simulink subsystem "Controller"  (R2020b)
settings: Solver=VariableStepAuto  StartTime=0.0  StopTime=10.0  RelTol=1e-3
values from neighbouring files (symbols this model uses):
  alpha = 0.5    [scratch.m]    (also in startup.m = 0.9)
  B = [-1,  0, 0, 0 ... (first row only)    [startup.m]
  g = 9.80665    [startup.m]
  leg_length = 1    [startup.m]
  leg_mass = 1.0    (= 1)    [startup.m]
  theta3_ref = -pi/4    (= -0.785398163397)    [scratch.m]    (also in startup.m = 0.785398163397)
  torso_length = 0.6    [startup.m]
  torso_mass = 1.0    (= 1)    [startup.m]
settings Model: Creator=PaulWintz  LastModifiedBy=PaulWintz

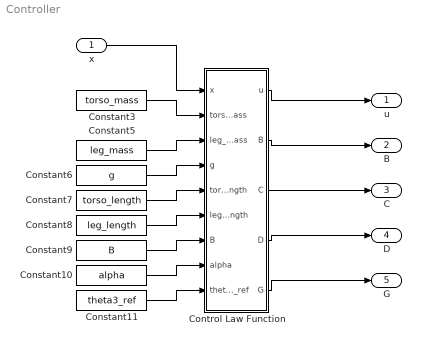
== system Controller ==
  x : Inport
  Constant10 : Constant  Value=alpha
  Constant11 : Constant  Value=theta3_ref
  Constant3 : Constant  Value=torso_mass
  Constant5 : Constant  Value=leg_mass
  Constant6 : Constant  Value=g
  Constant7 : Constant  Value=torso_length
  Constant8 : Constant  Value=leg_length
  Constant9 : Constant  Value=B
  Control Law Function : MATLAB Function  TreatAsAtomicUnit=on
  u : Outport
  B : Outport  Port=2
  C : Outport  Port=3
  D : Outport  Port=4
  G : Outport  Port=5
  wires:
  Constant10/1 -> Control Law Function/8(alpha)
  Constant3/1 -> Control Law Function/2(torso_mass)
  Constant6/1 -> Control Law Function/4(g)
  x/1 -> Control Law Function/1(x)
  Constant11/1 -> Control Law Function/9(theta3_ref)
  Constant5/1 -> Control Law Function/3(leg_mass)
  Constant7/1 -> Control Law Function/5(torso_length)
  Constant8/1 -> Control Law Function/6(leg_length)
  Constant9/1 -> Control Law Function/7("B ")
  Control Law Function/4(D) -> D/1
  Control Law Function/3(C) -> C/1
  Control Law Function/2(B) -> B/1
  Control Law Function/5(G) -> G/1
  Control Law Function/1(u) -> u/1

== matlab function Controller/Control Law Function ==
  settings: updateMethod=DISCRETE
  data: x input size=10; torso_mass input; u output; leg_mass input; g input; torso_length input; leg_length input; B input; alpha input; theta3_ref input; B output; C output; D output; G output
function [u, B, C, D, G] = control_law(x, torso_mass, leg_mass, g, torso_length, leg_length, B, alpha, theta3_ref)

    theta1 = x(1);
    theta2 = x(2);
    theta3 = x(3);
    theta4 = x(4);
    theta5 = x(5);
    omega1 = x(6);
    omega2 = x(7);
    omega3 = x(8);
    omega4 = x(9);
    omega5 = x(10);
    omega = x(6:10);
    
    m1 = leg_mass; %m1_sig
    m2 = leg_mass; %m2_sig
    m3 = leg_mass; %m3_sig
    m4 = leg_mass; %m4_sig
    m5 = torso_mass; %m5_sig
    
    L1 = leg_length; %L1_sig
    L2 = leg_length; %L2_sig
    L3 = leg_length; %L3_sig
    L4 = leg_length; %L4_sig
    L5 = torso_length; %L5_sig
  
    H = [1 0 0 0 0; 
         0 1 0 0 0; 
         0 0 1 0 0; 
         0 0 0 0 1];

    %hip_mass_sig is removed from the parameters of dynamic_matrices
    [C, D, G] = dynamic_matrices(x, g, torso_mass, leg_mass, leg_length, torso_length);

    y = [theta1;
        theta2;
        theta3-theta3_ref;
        theta5];
    Lf = [omega1; 
          omega2; 
          omega3; 
          omega5]; 
    LfLf = H * (D \ (-C*omega - G));
    LgLf = H * (D \ B);

    ydot = Lf;

    Psi = [psi_f([y(1); ydot(1)], alpha); 
           psi_f([y(2); ydot(2)], alpha); 
           psi_f([y(3); ydot(3)], alpha); 
           psi_f([y(4); ydot(4)], alpha)];
    u = LgLf \ (Psi - LfLf);

end

function y = phi(x, alpha_sig)
    y = x(1) + (1/2 - alpha_sig)*sign(x(2)).*abs(x(2)).^(2 - alpha_sig);
end

function y = psi_f(x, alpha_sig)
     y = -sign(x(2)).*abs(x(2)).^alpha_sig - sign(phi(x, alpha_sig)).*abs(phi(x, alpha_sig)).^(alpha_sig/(2-alpha_sig));
end

function [C, D, G] = dynamic_matrices(x, g, torso_mass, leg_mass, leg_length, torso_length)
                    %m1_sig, m2_sig, m3_sig, m4_sig, m5_sig, L1_sig, L2_sig, L3_sig, L4_sig, L5_sig

    theta1 = x(1);
    theta2 = x(2);
    theta3 = x(3);
    theta4 = x(4);
    theta5 = x(5);
    omega1 = x(6);
    omega2 = x(7);
    omega3 = x(8);
    omega4 = x(9);
    omega5 = x(10);
    
    %
    alpha10 = theta1;
    alpha20 = alpha10+theta2;
    alpha30 = alpha20+theta3;
    alpha40 = alpha30+theta4;
    alpha50 = alpha40+theta5;
    
    alpha21 = theta2;
    alpha31 = alpha21+theta3;
    alpha41 = alpha31+theta4;
    alpha51 = alpha21+theta5;
    
    alpha12 = -alpha21;
    alpha32 = theta3;
    alpha42 = alpha32+theta4;
    alpha52 = theta5;
    
    alpha13 = -alpha31;
    alpha23 = -alpha32;
    alpha43 = theta4;
    
    alpha14 = -alpha41;
    alpha24 = -alpha42;
    alpha34 = -alpha43;
    
    alpha15 = -alpha51;
    alpha25 = -alpha52;
    
    %R_22 = cos()
    
    R10_22 = cos(alpha10);
    R20_22 = cos(alpha20); 
    R30_22 = cos(alpha30); 
    R40_22 = cos(alpha40);
    R50_22 = cos(alpha50);
    
    R21_22 = cos(alpha21);
    R31_22 = cos(alpha31);
    R41_22 = cos(alpha41);
    R51_22 = cos(alpha51);
    
    R12_22 = cos(alpha12);
    R32_22 = cos(alpha32);
    R42_22 = cos(alpha42);
    R52_22 = cos(alpha52);
    
    R13_22 = cos(alpha13);
    R23_22 = cos(alpha23);
    R43_22 = cos(alpha43);
    
    R14_22 = cos(alpha14);
    R24_22 = cos(alpha24);
    R34_22 = cos(alpha34);
    
    R15_22 = cos(alpha15);
    R25_22 = cos(alpha25);
    
    %R_21 = sin()
    R21_21 = sin(alpha21);
    R31_21 = sin(alpha31);
    R41_21 = sin(alpha41);
    R51_21 = sin(alpha51);
    
    R12_21 = sin(alpha12);
    R32_21 = sin(alpha32);
    R42_21 = sin(alpha42);
    R52_21 = sin(alpha52);
    
    R13_21 = sin(alpha13);
    R23_21 = sin(alpha23);
    R43_21 = sin(alpha43);
    
    R14_21 = sin(alpha14);
    R24_21 = sin(alpha24);
    R34_21 = sin(alpha34);
    
    R15_21 = sin(alpha15);
    R25_21 = sin(alpha25);
    
    %I defined the masses and lengths in terms of leg_mass and
    %leg_length because they're already defined
    m1 = leg_mass; %m1_sig
    m2 = leg_mass; %m2_sig
    m3 = leg_mass; %m3_sig
    m4 = leg_mass; %m4_sig
    m5 = torso_mass; %m5_sig
    
    L1 = leg_length; %L1_sig
    L2 = leg_length; %L2_sig
    L3 = leg_length; %L3_sig
    L4 = leg_length; %L4_sig
    L5 = torso_length; %L5_sig   
    
    Pi = [(m1/4)+m2+m3+m4+m5, (m2+m3+m4+m5)*R12_22, (m3+m4)*R13_22, m4*R14_22, m5*R15_22;
        ((m2/2)+m3+m4+m5)*R21_22, m2/4+m3+m4+m5, (m3+m4)*R23_22, m4*R24_22, m5*R25_22;
        ((m3/2)+m4)*R31_22, ((m3/2)+m4)*R32_22, (m3/4)+m4, m4*R34_22, 0;
        m4/2*R41_22, m4/2*R42_22, m4/2*R43_22, m4/4, 0;
        m5/2*R51_22, m5/2*R52_22, 0, 0, m5/2];
    
    Lambda = [0, (m2+m3+m4+m5)*R12_21, (m3+m4)*R13_21, m4*R14_21, m5*R15_21;
        ((m2/2)+m3+m4+m5)*R21_21, 0, (m3+m4)*R23_21, m4*R24_21, m5*R25_21;
        ((m3/2)+m4)*R31_21, ((m3/2)+m4)*R32_21, 0, m4*R34_21, 0;
        m4/2*R41_21, m4/2*R42_21, m4/2*R43_21, 0, 0;
        m5/2*R51_21, m5/2*R52_21, 0, 0, 0];
    
    L = diag([L1, L2, L3, L4, L5]);
    
    G = g*[L1*(3/2*m1+m2+m3+m4+m5)*R10_22;
        L2*(3/2*m2+m3+m4+m5)*R20_22;
        L3*(3/2*m3+m4)*R30_22;
        3/2*L4*m4*R40_22;
        2*L5*m4*R50_22];
    
    D = L*Pi*L;
    C = -L*Lambda*L*diag([omega1, omega2, omega3, omega4, omega5]);

end
